simulink model "m_antifurto"  (Simulink 10.0)
settings: Solver=VariableStepDiscrete  StartTime=0.0  StopTime=0  FixedStep=1  RelTol=1e-3  AbsTol=1e-6  EnableMultiTasking=on
settings Model: Creator=prof. G. Celentano  LastModifiedBy=AR  ExtModeTrigMode=oneshot  ExtModeArmWhenConnect=off
settings SolverCC: AutoScaleAbsTol=off
settings DataIOCC: SignalLoggingSaveFormat=ModelDataLogs  SignalLoggingName=sigsOut
settings OptimizationCC: BooleanDataType=off  ExpressionDepthLimit=2147483647  InitFltsAndDblsToZero=on
settings DebuggingCC: SaveWithParameterizedLinksMsg=none  SignalResolutionControl=TryResolveAllWithWarning  MultiTaskDSMMsg=warning  MultiTaskCondExecSysMsg=none  FcnCallInpInsideContextMsg=warning  StateNameClashWarn=warning
settings HardwareCC: TargetUnknown=on
settings SFSimCC: SimUseLocalCustomCode=on  CustomCodeUndefinedFunction=FilterOut
settings RTWCC: RTWUseLocalCustomCode=on
settings GRTTargetCC: TargetFcnLib=ansi_tfl_tmw.mat

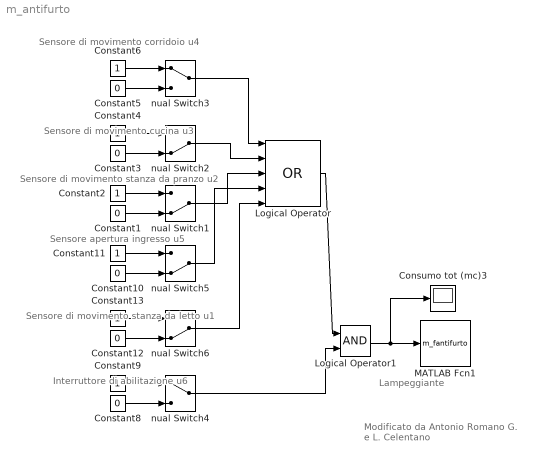
== system m_antifurto ==
  note: Interruttore di abilitazione u6
  note: Sensore apertura ingresso u5
  note: Sensore di movimento stanza da letto u1
  note: Lampeggiante
  note: Modificato da Antonio Romano
      | G. e L. Celentano
  note: Sensore di movimento stanza da pranzo u2
  note: Sensore di movimento cucina u3
  note: Sensore di movimento corridoio u4
  Constant{1,3,5,8,10,12} (6 alike) : Constant  Value=0
  Constant{2,4,6,9,11,13} (6 alike) : Constant
  Consumo tot (mc)3 : Display
  Logical Operator : Logic  Operator=OR  Inputs=5
  Logical Operator1 : Logic
  MATLAB Fcn1 : MATLABFcn  MATLABFcn=m_fantifurto  OutputDimensions=0
  nual Switch{1..2,5..6} (4 alike) : ManualSwitch  CurrentSetting=0
  nual Switch3 : ManualSwitch
  nual Switch4 : ManualSwitch
  wires:
  Logical Operator/1 -> Logical Operator1/1
  Constant13/1 -> nual Switch6/1
  Constant12/1 -> nual Switch6/2
  Constant9/1 -> nual Switch4/1
  Constant8/1 -> nual Switch4/2
  Constant11/1 -> nual Switch5/1
  Constant10/1 -> nual Switch5/2
  nual Switch6/1 -> Logical Operator/5
  nual Switch5/1 -> Logical Operator/4
  nual Switch4/1 -> Logical Operator1/2
  Logical Operator1/1 -> MATLAB Fcn1/1, Consumo tot (mc)3/1
  Constant2/1 -> nual Switch1/1
  Constant1/1 -> nual Switch1/2
  nual Switch1/1 -> Logical Operator/3
  nual Switch2/1 -> Logical Operator/2
  Constant4/1 -> nual Switch2/1
  Constant3/1 -> nual Switch2/2
  nual Switch3/1 -> Logical Operator/1
  Constant5/1 -> nual Switch3/2
  Constant6/1 -> nual Switch3/1
